simulink model "Wiper_system_Project"  (R2025b)
settings: Solver=FixedStepAuto  StartTime=0.0  StopTime=20  FixedStep=0.01  RelTol=1e-3
libraries: SignalEditorBlockLib x1, pil_lib x1
settings Model: Creator=Ahmed  LastModifiedBy=Ahmed
settings OptimizationCC: DefaultParameterBehavior=Inlined  UseDivisionForNetSlopeComputation=on  GainParamInheritBuiltInType=on  UseFloatMulNetSlope=on  InlineInvariantSignals=on  PassReuseOutputArgsAs=Individual arguments  ZeroExternalMemoryAtStartup=off  ZeroInternalMemoryAtStartup=off  NoFixptDivByZeroProtection=on  EfficientFloat2IntCast=on  LifeSpan=1  OptimizeBlockOrder=speed  DifferentSizesBufferReuse=on  EfficientTunableParamExpr=on
settings DebuggingCC: ParameterTunabilityLossMsg=error
settings HardwareCC: ProdLongLongMode=on
settings SFSimCC: MATLABDynamicMemAlloc=off
settings RTWCC: SystemTargetFile=ert.tlc  TemplateMakefile=ert_default_tmf  GenerateReport=on  LaunchReport=on  Description=Embedded Coder
settings CodeAppCC: ForceParamTrailComments=on  IgnoreCustomStorageClasses=off  OperatorAnnotations=on  SimulinkDataObjDesc=on  SFDataObjDesc=on  CustomSymbolStrGlobalVar=rt$N$M  CustomSymbolStrType=$N$M  CustomSymbolStrFcn=$N$M$F  CustomSymbolStrMacro=$N$M  InsertBlockDesc=on
settings ERTTargetCC: ERTCustomFileTemplate=example_file_process.tlc  ERTFilePackagingFormat=CompactWithDataFile  TargetLangStandard=C99 (ISO)  GenerateSampleERTMain=on  IncludeMdlTerminateFcn=off  CombineSignalStateStructs=on  SupportComplex=off  SupportContinuousTime=on

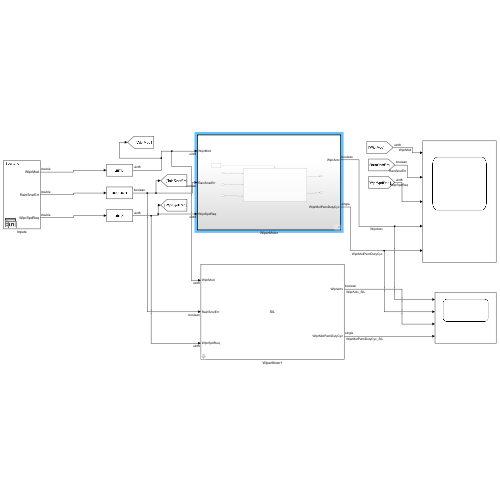
[thumbnail: Simulink's stored preview of the top-level diagram]
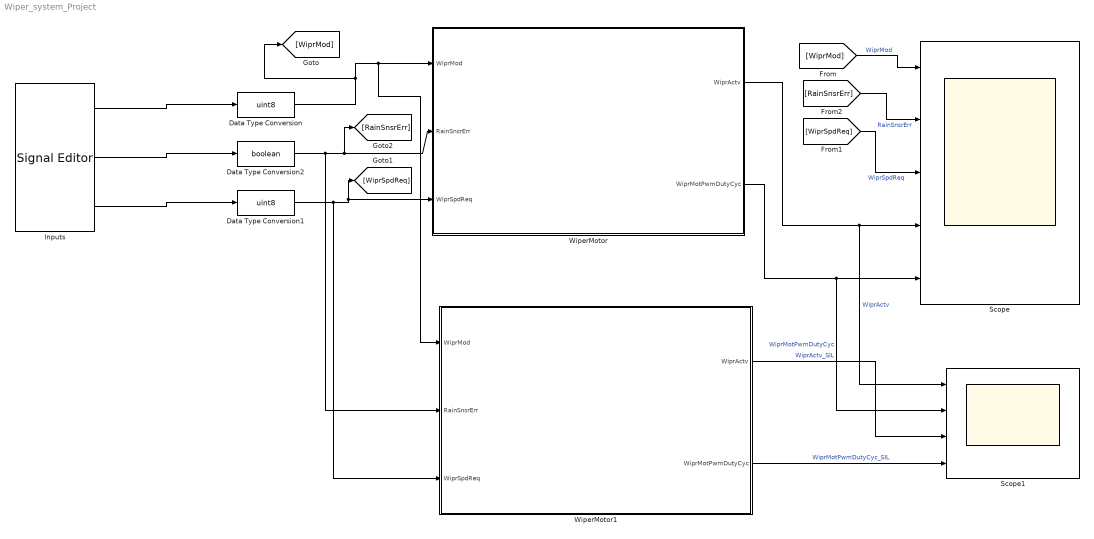
== system Wiper_system_Project ==
  Data Type Conversion : DataTypeConversion  OutDataTypeStr=uint8  SaturateOnIntegerOverflow=off  RndMeth=Floor
  Data Type Conversion1 : DataTypeConversion  OutDataTypeStr=uint8  SaturateOnIntegerOverflow=off  RndMeth=Floor
  Data Type Conversion2 : DataTypeConversion  OutDataTypeStr=boolean  SaturateOnIntegerOverflow=off  RndMeth=Floor
  Inputs : SignalEditorBlockLib/Signal Editor  FileName=Input_data_wiper.mat  ActiveScenario=Scenario  ActiveSignal=WiprMod  IsBus=off  OutputBusObjectStr=Bus: BusObject  SampleTime=0  ZeroCross=off  OutputAfterFinalValue=Setting to zero  Unit=inherit  PreserveSignalName=on  ApplySigPropsToAllScenarios=on  ApplySigPropsToAllSignals=off  SignalPropertySource=Dialog parameters
  Scope : Scope  NumInputPorts=5
      settings: ActiveDisplayYMinimum=-0.37499999999999989  ActiveDisplayYMaximum=3.375
  Scope1 : Scope  NumInputPorts=4
      settings: ActiveDisplayYMinimum=-0.12499999999999997  ActiveDisplayYMaximum=1.125
  WiperMotor : Subsystem  TreatAsAtomicUnit=on
  WiperMotor1 : Subsystem  Tag=__SL_testing_harness_stub_  DialogController=pil_create_dialog  LoadFcn=|
      | try
      |    if ~strcmp(rtw.pil.getPILVersion, '25.2 (R2025b)_15')
      |       set_param(gcb, 'DialogController', '');
      |       set_param(gcb, 'DialogControllerArgs', '');
      |    end
      | catch e
      |       set_param(gcb, 'DialogController', '');
      |       set_param(gcb, 'DialogControllerArgs', '');
      | end
      mask help: PIL:pil:XILBlockMaskDesc
      mask Display: disp('SIL');
  wires:
  Inputs/1 -> Data Type Conversion/1
  Inputs/3 -> Data Type Conversion1/1
  Data Type Conversion/1 -> [WiprMod], WiperMotor1/1(WiprMod), WiperMotor/1(WiprMod)
  Inputs/2 -> Data Type Conversion2/1
  Data Type Conversion1/1 -> WiperMotor1/3(WiprSpdReq), [WiprSpdReq], WiperMotor/3(WiprSpdReq)
  [WiprMod] -> Scope/1  "WiprMod"
  [RainSnsrErr] -> Scope/2  "RainSnsrErr"
  [WiprSpdReq] -> Scope/3  "WiprSpdReq"
  Data Type Conversion2/1 -> WiperMotor1/2(RainSnsrErr), WiperMotor/2(RainSnsrErr), [RainSnsrErr]
  WiperMotor/1(WiprActv) -> Scope1/1, Scope/4  "WiprActv"
  WiperMotor/2(WiprMotPwmDutyCyc) -> Scope1/2, Scope/5  "WiprMotPwmDutyCyc"
  WiperMotor1/1(WiprActv) -> Scope1/3  "WiprActv_SIL"
  WiperMotor1/2(WiprMotPwmDutyCyc) -> Scope1/4  "WiprMotPwmDutyCyc_SIL"

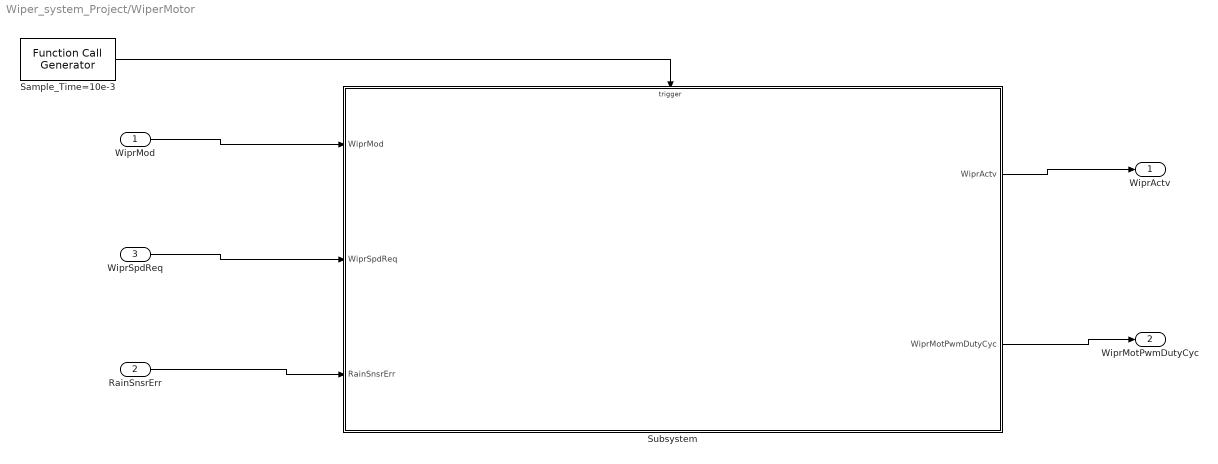
== system Wiper_system_Project/WiperMotor ==
  WiprMod : Inport  OutDataTypeStr=uint8
  RainSnsrErr : Inport  Port=2  OutDataTypeStr=boolean
  WiprSpdReq : Inport  Port=3  OutDataTypeStr=uint8
  Sample_Time=10e-3 : FunctionCallGenerator  SampleTime=10e-3
  Subsystem : Subsystem
  WiprActv : Outport
  WiprMotPwmDutyCyc : Outport  Port=2
  wires:
  WiprMod/1 -> Subsystem/1(WiprMod)
  WiprSpdReq/1 -> Subsystem/2(WiprSpdReq)
  RainSnsrErr/1 -> Subsystem/3(RainSnsrErr)
  Subsystem/1(WiprActv) -> WiprActv/1
  Subsystem/2(WiprMotPwmDutyCyc) -> WiprMotPwmDutyCyc/1
  Sample_Time=10e-3/1 -> Subsystem/Trigger

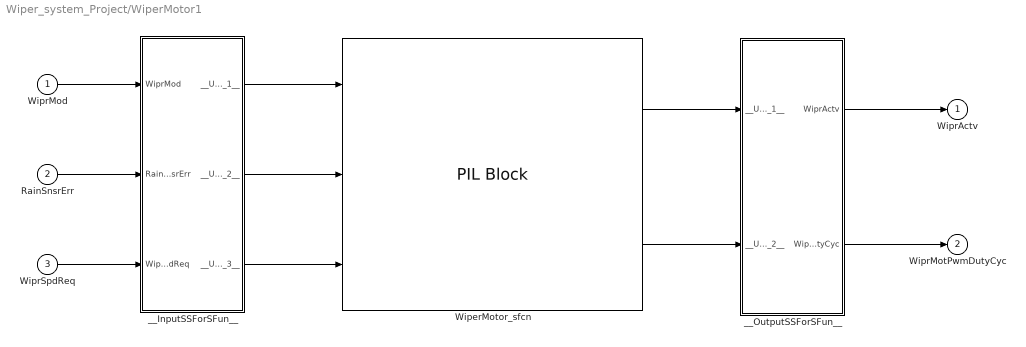
== system Wiper_system_Project/WiperMotor1 ==
  WiprMod : Inport  OutDataTypeStr=uint8
  RainSnsrErr : Inport  Port=2  OutDataTypeStr=boolean
  WiprSpdReq : Inport  Port=3  OutDataTypeStr=uint8
  WiperMotor_sfcn : pil_lib/PIL Block  SimulationMode=SIL  IsTopModelPIL=off  CodeDir=WiperMotor0_ert_rtw  AnchorDir=E:\PYthon_and_AI\Wiper_sys  ConfigName=Software-in-the-Loop (SIL)  XrelIsTopModelCode=on  XrelIsReusable=off  XrelDWorkNames={}  XrelDWorkTypes={}  XrelModelArgVals={}  XrelOrderedParamNames={}  XRelNonFiniteStyle=NONFINITE_UNUSED
  __InputSSForSFun__ : Subsystem
  __OutputSSForSFun__ : Subsystem
  WiprActv : Outport
  WiprMotPwmDutyCyc : Outport  Port=2
  wires:
  WiprMod/1 -> __InputSSForSFun__/1(WiprMod)
  RainSnsrErr/1 -> __InputSSForSFun__/2(RainSnsrErr)
  WiprSpdReq/1 -> __InputSSForSFun__/3(WiprSpdReq)
  __InputSSForSFun__/1(__UniqueOutportName__1__) -> WiperMotor_sfcn/1
  __InputSSForSFun__/2(__UniqueOutportName__2__) -> WiperMotor_sfcn/2
  __InputSSForSFun__/3(__UniqueOutportName__3__) -> WiperMotor_sfcn/3
  WiperMotor_sfcn/1 -> __OutputSSForSFun__/1(__UniqueInportName__1__)
  WiperMotor_sfcn/2 -> __OutputSSForSFun__/2(__UniqueInportName__2__)
  __OutputSSForSFun__/1(WiprActv) -> WiprActv/1
  __OutputSSForSFun__/2(WiprMotPwmDutyCyc) -> WiprMotPwmDutyCyc/1

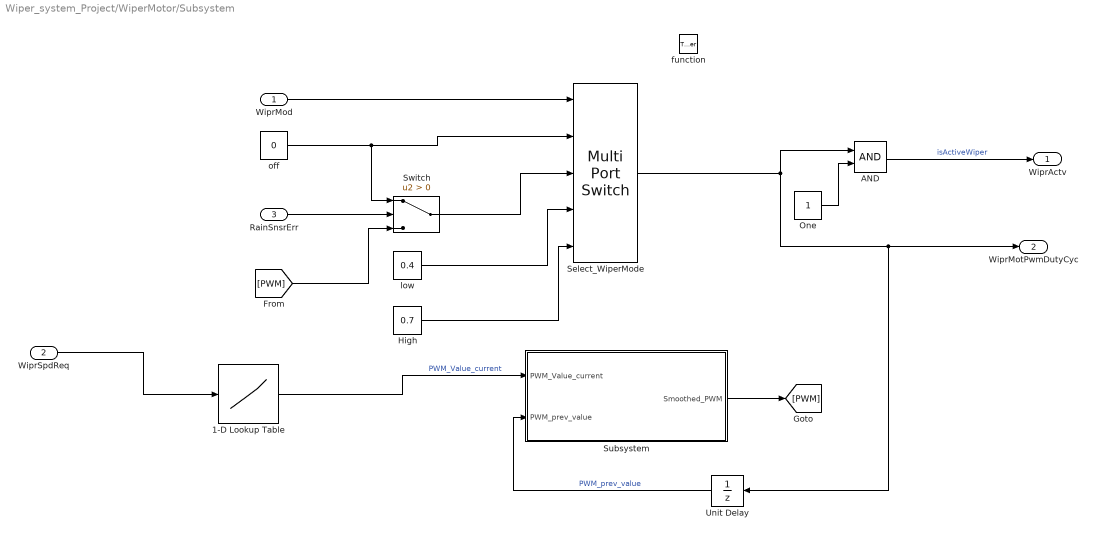
== system Wiper_system_Project/WiperMotor/Subsystem ==
  WiprMod : Inport
  WiprSpdReq : Inport  Port=2
  RainSnsrErr : Inport  Port=3
  function : TriggerPort  TriggerType=function-call  VariantControl=(inherit)
  1-D Lookup Table : Lookup_n-D  NumberOfTableDimensions=1  BreakpointsForDimension1=[0,1,2,3,4,5,6,7]  BreakpointsForDimension1DataTypeStr=single  Table=[0, 0.4, 0.45, 0.5, 0.55, 0.6, 0.65, 0.7]  TableDataTypeStr=single  ExtrapMethod=Clip  InternalRulePriority=Speed  OutDataTypeStr=single  RndMeth=Simplest
  AND : Logic  AllPortsSameDT=off  OutDataTypeStr=boolean
  High : Constant  Value=0.7  OutDataTypeStr=Inherit: Inherit via back propagation
  One : Constant  OutDataTypeStr=Inherit: Inherit via back propagation
  Select_WiperMode : MultiPortSwitch  DataPortOrder=Zero-based contiguous  Inputs=4  zeroidx=on  SaturateOnIntegerOverflow=off  InputSameDT=off
  Subsystem : Subsystem
  Switch : Switch  Criteria=u2 > Threshold  SaturateOnIntegerOverflow=off  InputSameDT=off
  Unit Delay : UnitDelay  SampleTime=-1  HasFrameUpgradeWarning=on
  low : Constant  Value=0.4  OutDataTypeStr=Inherit: Inherit via back propagation
  off : Constant  Value=0  OutDataTypeStr=Inherit: Inherit via back propagation
  WiprActv : Outport
  WiprMotPwmDutyCyc : Outport  Port=2
  wires:
  WiprMod/1 -> Select_WiperMode/1
  off/1 -> Switch/1, Select_WiperMode/2
  Switch/1 -> Select_WiperMode/3
  RainSnsrErr/1 -> Switch/2
  low/1 -> Select_WiperMode/4
  High/1 -> Select_WiperMode/5
  Select_WiperMode/1 -> Unit Delay/1, WiprMotPwmDutyCyc/1, AND/1
  One/1 -> AND/2
  AND/1 -> WiprActv/1  "isActiveWiper"
  Unit Delay/1 -> Subsystem/2(PWM_prev_value)  "PWM_prev_value"
  Subsystem/1(Smoothed_PWM) -> [PWM]
  [PWM] -> Switch/3
  WiprSpdReq/1 -> 1-D Lookup Table/1
  1-D Lookup Table/1 -> Subsystem/1(PWM_Value_current)  "PWM_Value_current"

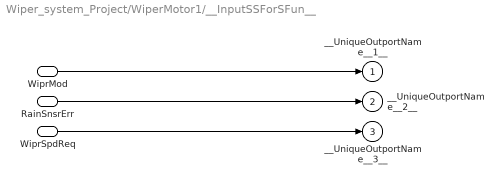
== system Wiper_system_Project/WiperMotor1/__InputSSForSFun__ ==
  WiprMod : Inport  OutDataTypeStr=uint8
  RainSnsrErr : Inport  Port=2  OutDataTypeStr=boolean
  WiprSpdReq : Inport  Port=3  OutDataTypeStr=uint8
  __UniqueOutportName__1__ : Outport
  __UniqueOutportName__2__ : Outport  Port=2
  __UniqueOutportName__3__ : Outport  Port=3
  wires:
  WiprMod/1 -> __UniqueOutportName__1__/1
  RainSnsrErr/1 -> __UniqueOutportName__2__/1
  WiprSpdReq/1 -> __UniqueOutportName__3__/1

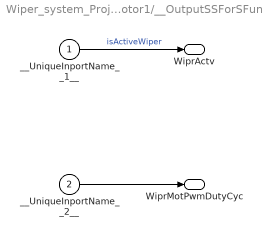
== system Wiper_system_Project/WiperMotor1/__OutputSSForSFun__ ==
  __UniqueInportName__1__ : Inport
  __UniqueInportName__2__ : Inport  Port=2
  WiprActv : Outport
  WiprMotPwmDutyCyc : Outport  Port=2
  wires:
  __UniqueInportName__1__/1 -> WiprActv/1  "isActiveWiper"
  __UniqueInportName__2__/1 -> WiprMotPwmDutyCyc/1

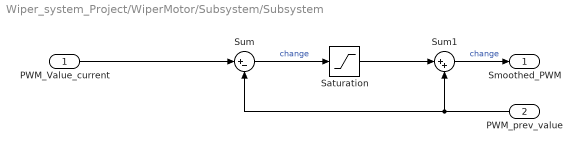
== system Wiper_system_Project/WiperMotor/Subsystem/Subsystem ==
  PWM_Value_current : Inport
  PWM_prev_value : Inport  Port=2
  Saturation : Saturate  UpperLimit=0.005  LowerLimit=-0.005
  Sum : Sum  Inputs=|+-
  Sum1 : Sum  Inputs=|++
  Smoothed_PWM : Outport
  wires:
  Sum/1 -> Saturation/1  "change"
  PWM_prev_value/1 -> Sum/2, Sum1/2
  PWM_Value_current/1 -> Sum/1
  Saturation/1 -> Sum1/1
  Sum1/1 -> Smoothed_PWM/1  "change"
